simulink library "csu_mnm_mems_noise_model_lib"  (R2014b)
settings: Solver=ode45  SolverMode=SingleTasking  StartTime=0.0  StopTime=10.0  RelTol=1e-3
values from neighbouring files (symbols this model uses):
  mnm_accel_bias_v = [0.1, -0.06, -0.05]    [csu_mnm_mems_noise_model_init.m]
  mnm_accel_noise_on = 1    [csu_mnm_mems_noise_model_init.m]
  mnm_accel_range = 16*9.81    (= 156.96)    [csu_mnm_mems_noise_model_init.m]
  mnm_accel_SF = 0*300/1e6    (= 0)    [csu_mnm_mems_noise_model_init.m]
  mnm_correlation_time = 100    [csu_mnm_mems_noise_model_init.m]
  mnm_dt = sim_time_step_size    [csu_mnm_mems_noise_model_init.m]
  mnm_gyro_bias_v = pi/180 * [-0.2, 0.12, 0.08]    [csu_mnm_mems_noise_model_init.m]
  mnm_gyro_g_sensitive = 2.471e-08 * [1 1 1]'    [csu_mnm_mems_noise_model_init.m]
  mnm_gyro_noise_on = 1    [csu_mnm_mems_noise_model_init.m]
  mnm_gyro_range = 250*pi/180    (= 4.36332312999)    [csu_mnm_mems_noise_model_init.m]
  mnm_gyro_SF = 100/1e6    (= 0.0001)    [csu_mnm_mems_noise_model_init.m]
  mnm_gyro_vibe_sensitive = 5.04e-09 * [1 1 1]'    [csu_mnm_mems_noise_model_init.m]
  mnm_thrust_accel_bias = [0.003 -0.002 -3.05]    [csu_mnm_mems_noise_model_init.m]
  mnm_thrust_accel_noise_factor = 25    [csu_mnm_mems_noise_model_init.m]
  mnm_thrust_gyro_noise_factor = 25    [csu_mnm_mems_noise_model_init.m]
undefined symbols (not defined in the file or in its folder): mnm_accel_noise_v, mnm_gyro_noise_v, my_accel_seed_v, my_gyro_seed_v, sim_time_step_size
undefined symbols (not defined in the file): my_accel_bias_seed_v, my_gyro_bias_seed_v
libraries: util_common_lib x3, simulink x1, util_info_lib x1
settings Model: Creator=hcannon  LastModifiedBy=mstewart

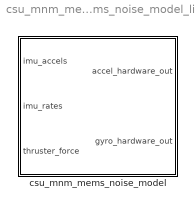
== system csu_mnm_mems_noise_model_lib ==
  csu_mnm_mems_noise_model : Subsystem  mask{accel_seed_v=my_accel_seed_v, accel_bias_seed_v=my_accel_bias_seed_v, gyro_seed_v=my_gyro_seed_v, gyro_bias_seed_v=my_gyro_bias_seed_v}
      mask prompts: accel_seed_v "Accel Output Noise Seed vector [1 x 3]"; accel_bias_seed_v "Accel Bias Noise Seed vector [1 x ]"; gyro_seed_v "Gyro Output Noise Seed vector [1 x 3]"; gyro_bias_seed_v "Gyro Bias Noise Seed vector [1 x 3]"

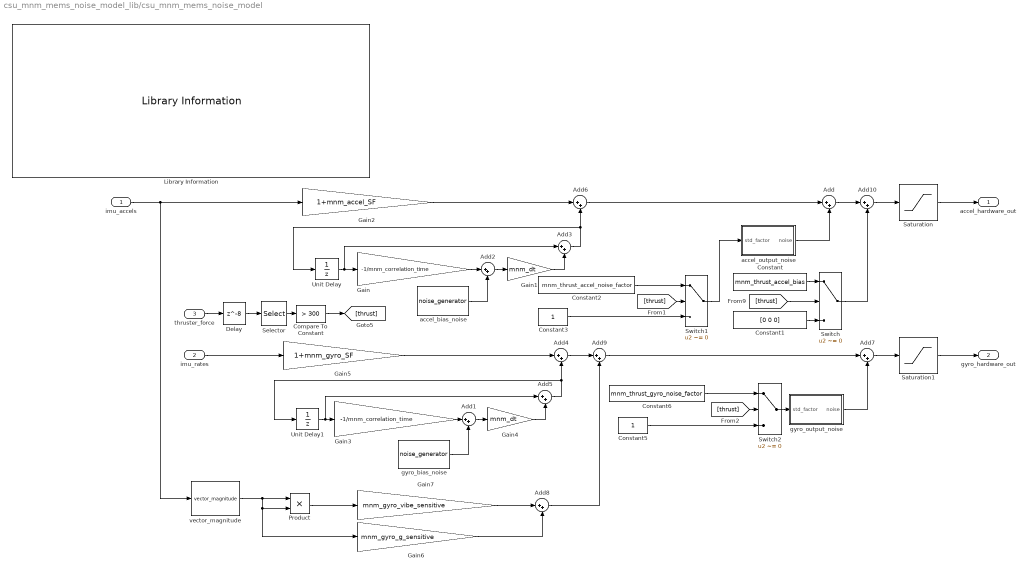
== system csu_mnm_mems_noise_model_lib/csu_mnm_mems_noise_model ==
  imu_accels : Inport
  imu_rates : Inport  Port=2
  thruster_force : Inport  Port=3
  Add{,1..10} (11 alike) : Sum  Inputs=|++
  Compare To Constant : simulink/Logic and Bit Operations/Compare To Constant  relop=>  const=300  OutDataTypeStr=boolean
  Constant : Constant  Value=mnm_thrust_accel_bias  OutDataTypeStr=double
  Constant1 : Constant  Value=[0 0 0]  OutDataTypeStr=double
  Constant2 : Constant  Value=mnm_thrust_accel_noise_factor  OutDataTypeStr=double
  Constant3 : Constant  OutDataTypeStr=double
  Constant5 : Constant  OutDataTypeStr=double
  Constant6 : Constant  Value=mnm_thrust_gyro_noise_factor  OutDataTypeStr=double
  Delay : Delay  DelayLength=8  InitialCondition=0
  Gain : Gain  Gain=-1/mnm_correlation_time
  Gain1 : Gain  Gain=mnm_dt
  Gain2 : Gain  Gain=1+mnm_accel_SF
  Gain3 : Gain  Gain=-1/mnm_correlation_time
  Gain4 : Gain  Gain=mnm_dt
  Gain5 : Gain  Gain=1+mnm_gyro_SF
  Gain6 : Gain  Gain=mnm_gyro_g_sensitive
  Gain7 : Gain  Gain=mnm_gyro_vibe_sensitive
  Library Information : util_info_lib/Library Information  owner='NONE'
  Product : Product  RndMeth=Zero
  Saturation : Saturate  UpperLimit=mnm_accel_range  LowerLimit=-mnm_accel_range
  Saturation1 : Saturate  UpperLimit=mnm_gyro_range  LowerLimit=-mnm_gyro_range
  Selector : Selector  InputPortWidth=3  Indices=[3]
  Switch : Switch  Criteria=u2 ~= 0
  Switch1 : Switch  Criteria=u2 ~= 0
  Switch2 : Switch  Criteria=u2 ~= 0
  Unit Delay : UnitDelay  SampleTime=-1
  Unit Delay1 : UnitDelay  SampleTime=-1
  accel_bias_noise : util_common_lib/noise_generator  std_dev=mnm_accel_bias_noise_v  bias=mnm_accel_bias_bias_v  seed=accel_bias_seed_v  on=mnm_accel_noise_on  sample_time=sim_time_step_size
  accel_output_noise : Subsystem
  gyro_bias_noise : util_common_lib/noise_generator  std_dev=mnm_gyro_bias_noise_v  bias=mnm_gyro_bias_bias_v  seed=gyro_bias_seed_v  on=mnm_gyro_noise_on  sample_time=sim_time_step_size
  gyro_output_noise : Subsystem
  vector_magnitude : util_common_lib/vector_magnitude  SystemSampleTime=-1
  accel_hardware_out : Outport
  gyro_hardware_out : Outport  Port=2
  wires:
  Switch1/1 -> accel_output_noise/1(std_factor)
  Selector/1 -> Compare To Constant/1
  Switch2/1 -> gyro_output_noise/1(std_factor)
  gyro_output_noise/1(noise) -> Add7/2
  Constant5/1 -> Switch2/3
  Constant6/1 -> Switch2/1
  [thrust] -> Switch2/2
  Constant3/1 -> Switch1/3
  Constant2/1 -> Switch1/1
  accel_output_noise/1(noise) -> Add/2
  [thrust] -> Switch1/2
  Compare To Constant/1 -> [thrust]
  thruster_force/1 -> Delay/1
  Switch/1 -> Add10/2
  Add/1 -> Add10/1
  Constant1/1 -> Switch/3
  Constant/1 -> Switch/1
  [thrust] -> Switch/2
  Saturation/1 -> accel_hardware_out/1
  Add10/1 -> Saturation/1
  Add8/1 -> Add9/2
  Add9/1 -> Add7/1
  Add4/1 -> Add9/1
  Gain6/1 -> Add8/2
  Gain7/1 -> Add8/1
  Product/1 -> Gain7/1
  vector_magnitude/1 -> Product/2, Gain6/1, Product/1
  Add6/1 -> Add/1
  Gain2/1 -> Add6/1
  Gain5/1 -> Add4/1
  Saturation1/1 -> gyro_hardware_out/1
  Add2/1 -> Gain1/1
  Gain1/1 -> Add3/2
  Unit Delay/1 -> Gain/1, Add3/1
  Add3/1 -> Add6/2, Unit Delay/1
  imu_accels/1 -> vector_magnitude/1, Gain2/1
  Gain/1 -> Add2/1
  accel_bias_noise/1 -> Add2/2
  Add1/1 -> Gain4/1
  Gain4/1 -> Add5/2
  Unit Delay1/1 -> Gain3/1, Add5/1
  Add5/1 -> Add4/2, Unit Delay1/1
  imu_rates/1 -> Gain5/1
  Gain3/1 -> Add1/1
  gyro_bias_noise/1 -> Add1/2
  Add7/1 -> Saturation1/1
  Delay/1 -> Selector/1

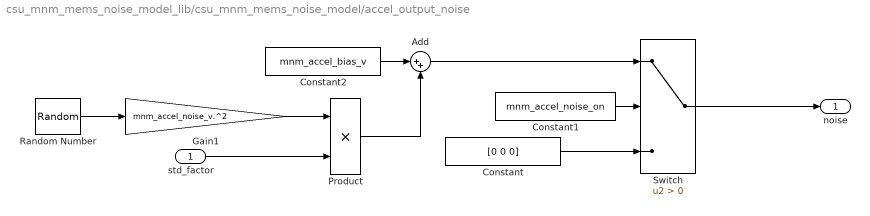
== system csu_mnm_mems_noise_model_lib/csu_mnm_mems_noise_model/accel_output_noise ==
  std_factor : Inport
  Add : Sum  Inputs=|++
  Constant : Constant  Value=[0 0 0]
  Constant1 : Constant  Value=mnm_accel_noise_on
  Constant2 : Constant  Value=mnm_accel_bias_v
  Gain1 : Gain  Gain=mnm_accel_noise_v.^2
  Product : Product
  Random Number : RandomNumber  Mean=[0 0 0]  Variance=[1 1 1]  Seed=my_accel_seed_v  SampleTime=sim_time_step_size
  Switch : Switch  Criteria=u2 > Threshold
  noise : Outport
  wires:
  std_factor/1 -> Product/2
  Gain1/1 -> Product/1
  Add/1 -> Switch/1
  Constant2/1 -> Add/1
  Product/1 -> Add/2
  Random Number/1 -> Gain1/1
  Constant1/1 -> Switch/2
  Constant/1 -> Switch/3
  Switch/1 -> noise/1

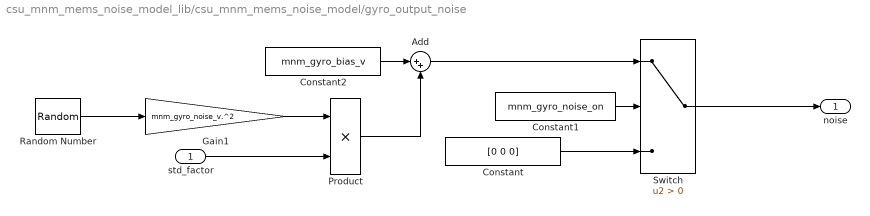
== system csu_mnm_mems_noise_model_lib/csu_mnm_mems_noise_model/gyro_output_noise ==
  std_factor : Inport
  Add : Sum  Inputs=|++
  Constant : Constant  Value=[0 0 0]
  Constant1 : Constant  Value=mnm_gyro_noise_on
  Constant2 : Constant  Value=mnm_gyro_bias_v
  Gain1 : Gain  Gain=mnm_gyro_noise_v.^2
  Product : Product
  Random Number : RandomNumber  Mean=[0 0 0]  Variance=[1 1 1]  Seed=my_gyro_seed_v  SampleTime=sim_time_step_size
  Switch : Switch  Criteria=u2 > Threshold
  noise : Outport
  wires:
  std_factor/1 -> Product/2
  Gain1/1 -> Product/1
  Add/1 -> Switch/1
  Constant2/1 -> Add/1
  Product/1 -> Add/2
  Random Number/1 -> Gain1/1
  Constant1/1 -> Switch/2
  Constant/1 -> Switch/3
  Switch/1 -> noise/1
